simulink model "ALL_JP360_DBW_V6_5_1103"  (R2022a)
settings: Solver=FixedStepAuto  StartTime=0.0  StopTime=inf  FixedStep=0.01  RelTol=1e-3  EnableMultiTasking=on
model workspace (MAT data in the model file):
  g = 9.8
undefined symbols (not defined in the file or in its folder): canChannel, delta_v_p, IPM_Line_C0, IPM_Line_C1, IPM_Line_C2, IPM_Line_C3, M, M_p, MRR_ObjDistX, MRR_ObjDistY, MRR_ObjFusionCamID, MRR_ObjFusionSig, MRR_ObjID, MRR_ObjRelVelX, MRR_ObjRelVelY, MRR_ObjType, MRR_ObjUpdFlg, none, obj_vaild, untracktime, V, videoinput
libraries: canfdmsglib x230, canfdlib x76, slpidlib x24, simulink x18, dspstat3 x14, ctrlSharedLib x1, simulink_extras x1, imaqlib x1, realtime_pacer_lib x1, dspvision x1, visionsinks x1
(part 47 of 55)

== system ALL_JP360_DBW_V6_5_1103/MsgFromCAN/VR_ADCU_MsgFromCAN/VR_ADCU_MRR_Obj_13_14_0x696 ==
  VR_ADCU_MRR_Obj_13_14_0x696FromInData : Inport  OutDataTypeStr=Bus:CAN_FD_MESSAGE_BUS
  Bus Creator : BusCreator  Inputs=30  OutDataTypeStr=Bus:VR_ADCU_MRR_Obj_13_14_0x696  NonVirtualBus=on
  CAN FD Unpack : canfdmsglib/CAN FD Unpack  CANdbFile=HiFire_T360_P789_1R1V_Pri_Matrix_CAN_V2.3_20220810.dbc  MsgList=(none)  MsgName=MRR_Obj_13_14_0x696  ProtocolMode=CAN FD  MsgIDType=Standard (11-bit identifier)  MsgIdentifier=1686  MsgLength=32  SignalInfo={'MRR_ObjDistX_13','26','12','BE','unsigned','Standard','0','0.0625','0','0','254.9375';'MRR_ObjDistX_14','130','12','BE','unsigned','Standard','0','0.0625','0','0','254.9375';'MRR_ObjDistY_13','44','14','BE','unsigned','Standard','0','0.0078125','-64','-64','63.9922';'MRR_ObjDistY_14','148','14','BE','unsigned','Standard','0','0.0078125','-64','-64','63.9922';'MRR_ObjExistProb_13','11','5','BE','unsigned','Standard','0','0.03125','0','0','0.96875';'MRR_ObjExistProb_14','115','5','BE','unsigned','Standard','0','0.03125','0','0','0.96875';'MRR_ObjFusionCamID_13','208','8','BE','unsigned','Standard','0','1','0','0','255';'MRR_ObjFusionCamID_14','216','8','BE','unsigned','Standard','0','1','0','0','255';'MRR_ObjFusionSig_13','98','2','BE','unsigned','Standard','0','1','0','0','3';'MRR_ObjFusionSig_14','202','2','BE','unsigned','Standard','0','1','0','0','3';'MRR_ObjID_13','0','8','BE','unsigned','Standard','0','1','0','0','255';'MRR_ObjID_14','104','8','BE','unsigned','Standard','0','1','0','0','255';'MRR_ObjMovingSts_13','103','3','BE','unsigned','Standard','0','1','0','0','7';'MRR_ObjMovingSts_14','207','3','BE','unsigned','Standard','0','1','0','0','7';'MRR_ObjObstacleProb_13','22','5','BE','unsigned','Standard','0','0.03125','0','0','0.96875';'MRR_ObjObstacleProb_14','126','5','BE','unsigned','Standard','0','0.03125','0','0','0.96875';'MRR_ObjRelAccelX_13','72','10','BE','unsigned','Standard','0','0.03125','-16','-16','15.9688';'MRR_ObjRelAccelX_14','176','10','BE','unsigned','Standard','0','0.03125','-16','-16','15.9688';'MRR_ObjRelAccelY_13','94','10','BE','unsigned','Standard','0','0.03125','-16','-16','15.9688';'MRR_ObjRelAccelY_14','198','10','BE','unsigned','Standard','0','0.03125','-16','-16','15.9688';'MRR_ObjRelVelX_13','63','13','BE','unsigned','Standard','0','0.03125','-128','-128','127.9688';'MRR_ObjRelVelX_14','167','13','BE','unsigned','Standard','0','0.03125','-128','-128','127.9688';'MRR_ObjRelVelY_13','66','13','BE','unsigned','Standard','0','0.03125','-128','-128','127.9688';'MRR_ObjRelVelY_14','170','13','BE','unsigned','Standard','0','0.03125','-128','-128','127.9688';'MRR_ObjType_13','90','4','BE','unsigned','Standard','0','1','0','0','15';'MRR_ObjType_14','194','4','BE','unsigned','Standard','0','1','0','0','15';'MRR_ObjUpdFlg_13','100','3','BE','unsigned','Standard','0','1','0','0','7';'MRR_ObjUpdFlg_14','204','3','BE','unsigned','Standard','0','1','0','0','7';'MRR_Obj_13_14_Checksum','248','16','BE','unsigned','Standard','0','1','0','0','65535';'MRR_Obj_13_14_MsgCounter','232','4','BE','unsigned','Standard','0','1','0','0','15'}  IDPort=off  TimestampPort=off  ErrorPort=off  RemotePort=off  LengthPort=off  StatusPort=off  BRSPort=off  ESIPort=off  DLCPort=off  ApplyMinMax=off
      settings: SourceProductBaseCode=ME,XP,VN  DataFormat=CANdb specified signals
  Data Type Conversion{1..6,15..24} (16 alike) : DataTypeConversion  OutDataTypeStr=single  SaturateOnIntegerOverflow=off  RndMeth=Floor
  Data Type Conversion{9..10,13..14,25..28,30} (9 alike) : DataTypeConversion  OutDataTypeStr=int8  SaturateOnIntegerOverflow=off  RndMeth=Floor
  Data Type Conversion{7..8,11..12} (4 alike) : DataTypeConversion  OutDataTypeStr=uint8  SaturateOnIntegerOverflow=off  RndMeth=Floor
  Data Type Conversion29 : DataTypeConversion  OutDataTypeStr=uint16  SaturateOnIntegerOverflow=off  RndMeth=Floor
  VR_ADCU_MRR_Obj_13_14_0x696FromOutData : Outport  OutDataTypeStr=Bus:VR_ADCU_MRR_Obj_13_14_0x696
  wires:
  CAN FD Unpack/1 -> Data Type Conversion1/1
  CAN FD Unpack/2 -> Data Type Conversion2/1
  CAN FD Unpack/3 -> Data Type Conversion3/1
  CAN FD Unpack/4 -> Data Type Conversion4/1
  CAN FD Unpack/5 -> Data Type Conversion5/1
  CAN FD Unpack/6 -> Data Type Conversion6/1
  CAN FD Unpack/7 -> Data Type Conversion7/1
  CAN FD Unpack/8 -> Data Type Conversion8/1
  CAN FD Unpack/9 -> Data Type Conversion9/1
  CAN FD Unpack/10 -> Data Type Conversion10/1
  CAN FD Unpack/11 -> Data Type Conversion11/1
  CAN FD Unpack/12 -> Data Type Conversion12/1
  CAN FD Unpack/13 -> Data Type Conversion13/1
  CAN FD Unpack/14 -> Data Type Conversion14/1
  CAN FD Unpack/15 -> Data Type Conversion15/1
  CAN FD Unpack/16 -> Data Type Conversion16/1
  CAN FD Unpack/17 -> Data Type Conversion17/1
  CAN FD Unpack/18 -> Data Type Conversion18/1
  CAN FD Unpack/19 -> Data Type Conversion19/1
  CAN FD Unpack/20 -> Data Type Conversion20/1
  CAN FD Unpack/21 -> Data Type Conversion21/1
  CAN FD Unpack/22 -> Data Type Conversion22/1
  CAN FD Unpack/23 -> Data Type Conversion23/1
  CAN FD Unpack/24 -> Data Type Conversion24/1
  CAN FD Unpack/25 -> Data Type Conversion25/1
  CAN FD Unpack/26 -> Data Type Conversion26/1
  CAN FD Unpack/27 -> Data Type Conversion27/1
  CAN FD Unpack/28 -> Data Type Conversion28/1
  CAN FD Unpack/29 -> Data Type Conversion29/1
  CAN FD Unpack/30 -> Data Type Conversion30/1
  Data Type Conversion1/1 -> Bus Creator/1  "MRR_ObjDistX_13"
  Data Type Conversion2/1 -> Bus Creator/2  "MRR_ObjDistX_14"
  Data Type Conversion3/1 -> Bus Creator/3  "MRR_ObjDistY_13"
  Data Type Conversion4/1 -> Bus Creator/4  "MRR_ObjDistY_14"
  Data Type Conversion5/1 -> Bus Creator/5  "MRR_ObjExistProb_13"
  Data Type Conversion6/1 -> Bus Creator/6  "MRR_ObjExistProb_14"
  Data Type Conversion7/1 -> Bus Creator/7  "MRR_ObjFusionCamID_13"
  Data Type Conversion8/1 -> Bus Creator/8  "MRR_ObjFusionCamID_14"
  Data Type Conversion9/1 -> Bus Creator/9  "MRR_ObjFusionSig_13"
  Data Type Conversion10/1 -> Bus Creator/10  "MRR_ObjFusionSig_14"
  Data Type Conversion11/1 -> Bus Creator/11  "MRR_ObjID_13"
  Data Type Conversion12/1 -> Bus Creator/12  "MRR_ObjID_14"
  Data Type Conversion13/1 -> Bus Creator/13  "MRR_ObjMovingSts_13"
  Data Type Conversion14/1 -> Bus Creator/14  "MRR_ObjMovingSts_14"
  Data Type Conversion15/1 -> Bus Creator/15  "MRR_ObjObstacleProb_13"
  Data Type Conversion16/1 -> Bus Creator/16  "MRR_ObjObstacleProb_14"
  Data Type Conversion17/1 -> Bus Creator/17  "MRR_ObjRelAccelX_13"
  Data Type Conversion18/1 -> Bus Creator/18  "MRR_ObjRelAccelX_14"
  Data Type Conversion19/1 -> Bus Creator/19  "MRR_ObjRelAccelY_13"
  Data Type Conversion20/1 -> Bus Creator/20  "MRR_ObjRelAccelY_14"
  Data Type Conversion21/1 -> Bus Creator/21  "MRR_ObjRelVelX_13"
  Data Type Conversion22/1 -> Bus Creator/22  "MRR_ObjRelVelX_14"
  Data Type Conversion23/1 -> Bus Creator/23  "MRR_ObjRelVelY_13"
  Data Type Conversion24/1 -> Bus Creator/24  "MRR_ObjRelVelY_14"
  Data Type Conversion25/1 -> Bus Creator/25  "MRR_ObjType_13"
  Data Type Conversion26/1 -> Bus Creator/26  "MRR_ObjType_14"
  Data Type Conversion27/1 -> Bus Creator/27  "MRR_ObjUpdFlg_13"
  Data Type Conversion28/1 -> Bus Creator/28  "MRR_ObjUpdFlg_14"
  Data Type Conversion29/1 -> Bus Creator/29  "MRR_Obj_13_14_Checksum"
  Data Type Conversion30/1 -> Bus Creator/30  "MRR_Obj_13_14_MsgCounter"
  Bus Creator/1 -> VR_ADCU_MRR_Obj_13_14_0x696FromOutData/1  "VR_ADCU_MRR_Obj_13_14_0x696FromOutData"
  VR_ADCU_MRR_Obj_13_14_0x696FromInData/1 -> CAN FD Unpack/1  "VR_ADCU_MRR_Obj_13_14_0x696FromInData"

== system ALL_JP360_DBW_V6_5_1103/MsgFromCAN/VR_ADCU_MsgFromCAN/VR_ADCU_MRR_Obj_15_16_0x697 ==
  VR_ADCU_MRR_Obj_15_16_0x697FromInData : Inport  OutDataTypeStr=Bus:CAN_FD_MESSAGE_BUS
  Bus Creator : BusCreator  Inputs=30  OutDataTypeStr=Bus:VR_ADCU_MRR_Obj_15_16_0x697  NonVirtualBus=on
  CAN FD Unpack : canfdmsglib/CAN FD Unpack  CANdbFile=HiFire_T360_P789_1R1V_Pri_Matrix_CAN_V2.3_20220810.dbc  MsgList=(none)  MsgName=MRR_Obj_15_16_0x697  ProtocolMode=CAN FD  MsgIDType=Standard (11-bit identifier)  MsgIdentifier=1687  MsgLength=32  SignalInfo={'MRR_ObjDistX_15','26','12','BE','unsigned','Standard','0','0.0625','0','0','254.9375';'MRR_ObjDistX_16','130','12','BE','unsigned','Standard','0','0.0625','0','0','254.9375';'MRR_ObjDistY_15','44','14','BE','unsigned','Standard','0','0.0078125','-64','-64','63.9922';'MRR_ObjDistY_16','148','14','BE','unsigned','Standard','0','0.0078125','-64','-64','63.9922';'MRR_ObjExistProb_15','11','5','BE','unsigned','Standard','0','0.03125','0','0','0.96875';'MRR_ObjExistProb_16','115','5','BE','unsigned','Standard','0','0.03125','0','0','0.96875';'MRR_ObjFusionCamID_15','208','8','BE','unsigned','Standard','0','1','0','0','255';'MRR_ObjFusionCamID_16','216','8','BE','unsigned','Standard','0','1','0','0','255';'MRR_ObjFusionSig_15','98','2','BE','unsigned','Standard','0','1','0','0','3';'MRR_ObjFusionSig_16','202','2','BE','unsigned','Standard','0','1','0','0','3';'MRR_ObjID_15','0','8','BE','unsigned','Standard','0','1','0','0','255';'MRR_ObjID_16','104','8','BE','unsigned','Standard','0','1','0','0','255';'MRR_ObjMovingSts_15','103','3','BE','unsigned','Standard','0','1','0','0','7';'MRR_ObjMovingSts_16','207','3','BE','unsigned','Standard','0','1','0','0','7';'MRR_ObjObstacleProb_15','22','5','BE','unsigned','Standard','0','0.03125','0','0','0.96875';'MRR_ObjObstacleProb_16','126','5','BE','unsigned','Standard','0','0.03125','0','0','0.96875';'MRR_ObjRelAccelX_15','72','10','BE','unsigned','Standard','0','0.03125','-16','-16','15.9688';'MRR_ObjRelAccelX_16','176','10','BE','unsigned','Standard','0','0.03125','-16','-16','15.9688';'MRR_ObjRelAccelY_15','94','10','BE','unsigned','Standard','0','0.03125','-16','-16','15.9688';'MRR_ObjRelAccelY_16','198','10','BE','unsigned','Standard','0','0.03125','-16','-16','15.9688';'MRR_ObjRelVelX_15','63','13','BE','unsigned','Standard','0','0.03125','-128','-128','127.9688';'MRR_ObjRelVelX_16','167','13','BE','unsigned','Standard','0','0.03125','-128','-128','127.9688';'MRR_ObjRelVelY_15','66','13','BE','unsigned','Standard','0','0.03125','-128','-128','127.9688';'MRR_ObjRelVelY_16','170','13','BE','unsigned','Standard','0','0.03125','-128','-128','127.9688';'MRR_ObjType_15','90','4','BE','unsigned','Standard','0','1','0','0','15';'MRR_ObjType_16','194','4','BE','unsigned','Standard','0','1','0','0','15';'MRR_ObjUpdFlg_15','100','3','BE','unsigned','Standard','0','1','0','0','7';'MRR_ObjUpdFlg_16','204','3','BE','unsigned','Standard','0','1','0','0','7';'MRR_Obj_15_16_Checksum','248','16','BE','unsigned','Standard','0','1','0','0','65535';'MRR_Obj_15_16_MsgCounter','232','4','BE','unsigned','Standard','0','1','0','0','15'}  IDPort=off  TimestampPort=off  ErrorPort=off  RemotePort=off  LengthPort=off  StatusPort=off  BRSPort=off  ESIPort=off  DLCPort=off  ApplyMinMax=off
      settings: SourceProductBaseCode=ME,XP,VN  DataFormat=CANdb specified signals
  Data Type Conversion{1..6,15..24} (16 alike) : DataTypeConversion  OutDataTypeStr=single  SaturateOnIntegerOverflow=off  RndMeth=Floor
  Data Type Conversion{9..10,13..14,25..28,30} (9 alike) : DataTypeConversion  OutDataTypeStr=int8  SaturateOnIntegerOverflow=off  RndMeth=Floor
  Data Type Conversion{7..8,11..12} (4 alike) : DataTypeConversion  OutDataTypeStr=uint8  SaturateOnIntegerOverflow=off  RndMeth=Floor
  Data Type Conversion29 : DataTypeConversion  OutDataTypeStr=uint16  SaturateOnIntegerOverflow=off  RndMeth=Floor
  VR_ADCU_MRR_Obj_15_16_0x697FromOutData : Outport  OutDataTypeStr=Bus:VR_ADCU_MRR_Obj_15_16_0x697
  wires:
  CAN FD Unpack/1 -> Data Type Conversion1/1
  CAN FD Unpack/2 -> Data Type Conversion2/1
  CAN FD Unpack/3 -> Data Type Conversion3/1
  CAN FD Unpack/4 -> Data Type Conversion4/1
  CAN FD Unpack/5 -> Data Type Conversion5/1
  CAN FD Unpack/6 -> Data Type Conversion6/1
  CAN FD Unpack/7 -> Data Type Conversion7/1
  CAN FD Unpack/8 -> Data Type Conversion8/1
  CAN FD Unpack/9 -> Data Type Conversion9/1
  CAN FD Unpack/10 -> Data Type Conversion10/1
  CAN FD Unpack/11 -> Data Type Conversion11/1
  CAN FD Unpack/12 -> Data Type Conversion12/1
  CAN FD Unpack/13 -> Data Type Conversion13/1
  CAN FD Unpack/14 -> Data Type Conversion14/1
  CAN FD Unpack/15 -> Data Type Conversion15/1
  CAN FD Unpack/16 -> Data Type Conversion16/1
  CAN FD Unpack/17 -> Data Type Conversion17/1
  CAN FD Unpack/18 -> Data Type Conversion18/1
  CAN FD Unpack/19 -> Data Type Conversion19/1
  CAN FD Unpack/20 -> Data Type Conversion20/1
  CAN FD Unpack/21 -> Data Type Conversion21/1
  CAN FD Unpack/22 -> Data Type Conversion22/1
  CAN FD Unpack/23 -> Data Type Conversion23/1
  CAN FD Unpack/24 -> Data Type Conversion24/1
  CAN FD Unpack/25 -> Data Type Conversion25/1
  CAN FD Unpack/26 -> Data Type Conversion26/1
  CAN FD Unpack/27 -> Data Type Conversion27/1
  CAN FD Unpack/28 -> Data Type Conversion28/1
  CAN FD Unpack/29 -> Data Type Conversion29/1
  CAN FD Unpack/30 -> Data Type Conversion30/1
  Data Type Conversion1/1 -> Bus Creator/1  "MRR_ObjDistX_15"
  Data Type Conversion2/1 -> Bus Creator/2  "MRR_ObjDistX_16"
  Data Type Conversion3/1 -> Bus Creator/3  "MRR_ObjDistY_15"
  Data Type Conversion4/1 -> Bus Creator/4  "MRR_ObjDistY_16"
  Data Type Conversion5/1 -> Bus Creator/5  "MRR_ObjExistProb_15"
  Data Type Conversion6/1 -> Bus Creator/6  "MRR_ObjExistProb_16"
  Data Type Conversion7/1 -> Bus Creator/7  "MRR_ObjFusionCamID_15"
  Data Type Conversion8/1 -> Bus Creator/8  "MRR_ObjFusionCamID_16"
  Data Type Conversion9/1 -> Bus Creator/9  "MRR_ObjFusionSig_15"
  Data Type Conversion10/1 -> Bus Creator/10  "MRR_ObjFusionSig_16"
  Data Type Conversion11/1 -> Bus Creator/11  "MRR_ObjID_15"
  Data Type Conversion12/1 -> Bus Creator/12  "MRR_ObjID_16"
  Data Type Conversion13/1 -> Bus Creator/13  "MRR_ObjMovingSts_15"
  Data Type Conversion14/1 -> Bus Creator/14  "MRR_ObjMovingSts_16"
  Data Type Conversion15/1 -> Bus Creator/15  "MRR_ObjObstacleProb_15"
  Data Type Conversion16/1 -> Bus Creator/16  "MRR_ObjObstacleProb_16"
  Data Type Conversion17/1 -> Bus Creator/17  "MRR_ObjRelAccelX_15"
  Data Type Conversion18/1 -> Bus Creator/18  "MRR_ObjRelAccelX_16"
  Data Type Conversion19/1 -> Bus Creator/19  "MRR_ObjRelAccelY_15"
  Data Type Conversion20/1 -> Bus Creator/20  "MRR_ObjRelAccelY_16"
  Data Type Conversion21/1 -> Bus Creator/21  "MRR_ObjRelVelX_15"
  Data Type Conversion22/1 -> Bus Creator/22  "MRR_ObjRelVelX_16"
  Data Type Conversion23/1 -> Bus Creator/23  "MRR_ObjRelVelY_15"
  Data Type Conversion24/1 -> Bus Creator/24  "MRR_ObjRelVelY_16"
  Data Type Conversion25/1 -> Bus Creator/25  "MRR_ObjType_15"
  Data Type Conversion26/1 -> Bus Creator/26  "MRR_ObjType_16"
  Data Type Conversion27/1 -> Bus Creator/27  "MRR_ObjUpdFlg_15"
  Data Type Conversion28/1 -> Bus Creator/28  "MRR_ObjUpdFlg_16"
  Data Type Conversion29/1 -> Bus Creator/29  "MRR_Obj_15_16_Checksum"
  Data Type Conversion30/1 -> Bus Creator/30  "MRR_Obj_15_16_MsgCounter"
  Bus Creator/1 -> VR_ADCU_MRR_Obj_15_16_0x697FromOutData/1  "VR_ADCU_MRR_Obj_15_16_0x697FromOutData"
  VR_ADCU_MRR_Obj_15_16_0x697FromInData/1 -> CAN FD Unpack/1  "VR_ADCU_MRR_Obj_15_16_0x697FromInData"

== system ALL_JP360_DBW_V6_5_1103/MsgFromCAN/VR_ADCU_MsgFromCAN/VR_ADCU_MRR_Obj_17_18_0x698 ==
  VR_ADCU_MRR_Obj_17_18_0x698FromInData : Inport  OutDataTypeStr=Bus:CAN_FD_MESSAGE_BUS
  Bus Creator : BusCreator  Inputs=30  OutDataTypeStr=Bus:VR_ADCU_MRR_Obj_17_18_0x698  NonVirtualBus=on
  CAN FD Unpack : canfdmsglib/CAN FD Unpack  CANdbFile=HiFire_T360_P789_1R1V_Pri_Matrix_CAN_V2.3_20220810.dbc  MsgList=(none)  MsgName=MRR_Obj_17_18_0x698  ProtocolMode=CAN FD  MsgIDType=Standard (11-bit identifier)  MsgIdentifier=1688  MsgLength=32  SignalInfo={'MRR_ObjDistX_17','26','12','BE','unsigned','Standard','0','0.0625','0','0','254.9375';'MRR_ObjDistX_18','130','12','BE','unsigned','Standard','0','0.0625','0','0','254.9375';'MRR_ObjDistY_17','44','14','BE','unsigned','Standard','0','0.0078125','-64','-64','63.9922';'MRR_ObjDistY_18','148','14','BE','unsigned','Standard','0','0.0078125','-64','-64','63.9922';'MRR_ObjExistProb_17','11','5','BE','unsigned','Standard','0','0.03125','0','0','0.96875';'MRR_ObjExistProb_18','115','5','BE','unsigned','Standard','0','0.03125','0','0','0.96875';'MRR_ObjFusionCamID_17','208','8','BE','unsigned','Standard','0','1','0','0','255';'MRR_ObjFusionCamID_18','216','8','BE','unsigned','Standard','0','1','0','0','255';'MRR_ObjFusionSig_17','98','2','BE','unsigned','Standard','0','1','0','0','3';'MRR_ObjFusionSig_18','202','2','BE','unsigned','Standard','0','1','0','0','3';'MRR_ObjID_17','0','8','BE','unsigned','Standard','0','1','0','0','255';'MRR_ObjID_18','104','8','BE','unsigned','Standard','0','1','0','0','255';'MRR_ObjMovingSts_17','103','3','BE','unsigned','Standard','0','1','0','0','7';'MRR_ObjMovingSts_18','207','3','BE','unsigned','Standard','0','1','0','0','7';'MRR_ObjObstacleProb_17','22','5','BE','unsigned','Standard','0','0.03125','0','0','0.96875';'MRR_ObjObstacleProb_18','126','5','BE','unsigned','Standard','0','0.03125','0','0','0.96875';'MRR_ObjRelAccelX_17','72','10','BE','unsigned','Standard','0','0.03125','-16','-16','15.9688';'MRR_ObjRelAccelX_18','176','10','BE','unsigned','Standard','0','0.03125','-16','-16','15.9688';'MRR_ObjRelAccelY_17','94','10','BE','unsigned','Standard','0','0.03125','-16','-16','15.9688';'MRR_ObjRelAccelY_18','198','10','BE','unsigned','Standard','0','0.03125','-16','-16','15.9688';'MRR_ObjRelVelX_17','63','13','BE','unsigned','Standard','0','0.03125','-128','-128','127.9688';'MRR_ObjRelVelX_18','167','13','BE','unsigned','Standard','0','0.03125','-128','-128','127.9688';'MRR_ObjRelVelY_17','66','13','BE','unsigned','Standard','0','0.03125','-128','-128','127.9688';'MRR_ObjRelVelY_18','170','13','BE','unsigned','Standard','0','0.03125','-128','-128','127.9688';'MRR_ObjType_17','90','4','BE','unsigned','Standard','0','1','0','0','15';'MRR_ObjType_18','194','4','BE','unsigned','Standard','0','1','0','0','15';'MRR_ObjUpdFlg_17','100','3','BE','unsigned','Standard','0','1','0','0','7';'MRR_ObjUpdFlg_18','204','3','BE','unsigned','Standard','0','1','0','0','7';'MRR_Obj_17_18_Checksum','248','16','BE','unsigned','Standard','0','1','0','0','65535';'MRR_Obj_17_18_MsgCounter','232','4','BE','unsigned','Standard','0','1','0','0','15'}  IDPort=off  TimestampPort=off  ErrorPort=off  RemotePort=off  LengthPort=off  StatusPort=off  BRSPort=off  ESIPort=off  DLCPort=off  ApplyMinMax=off
      settings: SourceProductBaseCode=ME,XP,VN  DataFormat=CANdb specified signals
  Data Type Conversion{1..6,15..24} (16 alike) : DataTypeConversion  OutDataTypeStr=single  SaturateOnIntegerOverflow=off  RndMeth=Floor
  Data Type Conversion{9..10,13..14,25..28,30} (9 alike) : DataTypeConversion  OutDataTypeStr=int8  SaturateOnIntegerOverflow=off  RndMeth=Floor
  Data Type Conversion{7..8,11..12} (4 alike) : DataTypeConversion  OutDataTypeStr=uint8  SaturateOnIntegerOverflow=off  RndMeth=Floor
  Data Type Conversion29 : DataTypeConversion  OutDataTypeStr=uint16  SaturateOnIntegerOverflow=off  RndMeth=Floor
  VR_ADCU_MRR_Obj_17_18_0x698FromOutData : Outport  OutDataTypeStr=Bus:VR_ADCU_MRR_Obj_17_18_0x698
  wires:
  CAN FD Unpack/1 -> Data Type Conversion1/1
  CAN FD Unpack/2 -> Data Type Conversion2/1
  CAN FD Unpack/3 -> Data Type Conversion3/1
  CAN FD Unpack/4 -> Data Type Conversion4/1
  CAN FD Unpack/5 -> Data Type Conversion5/1
  CAN FD Unpack/6 -> Data Type Conversion6/1
  CAN FD Unpack/7 -> Data Type Conversion7/1
  CAN FD Unpack/8 -> Data Type Conversion8/1
  CAN FD Unpack/9 -> Data Type Conversion9/1
  CAN FD Unpack/10 -> Data Type Conversion10/1
  CAN FD Unpack/11 -> Data Type Conversion11/1
  CAN FD Unpack/12 -> Data Type Conversion12/1
  CAN FD Unpack/13 -> Data Type Conversion13/1
  CAN FD Unpack/14 -> Data Type Conversion14/1
  CAN FD Unpack/15 -> Data Type Conversion15/1
  CAN FD Unpack/16 -> Data Type Conversion16/1
  CAN FD Unpack/17 -> Data Type Conversion17/1
  CAN FD Unpack/18 -> Data Type Conversion18/1
  CAN FD Unpack/19 -> Data Type Conversion19/1
  CAN FD Unpack/20 -> Data Type Conversion20/1
  CAN FD Unpack/21 -> Data Type Conversion21/1
  CAN FD Unpack/22 -> Data Type Conversion22/1
  CAN FD Unpack/23 -> Data Type Conversion23/1
  CAN FD Unpack/24 -> Data Type Conversion24/1
  CAN FD Unpack/25 -> Data Type Conversion25/1
  CAN FD Unpack/26 -> Data Type Conversion26/1
  CAN FD Unpack/27 -> Data Type Conversion27/1
  CAN FD Unpack/28 -> Data Type Conversion28/1
  CAN FD Unpack/29 -> Data Type Conversion29/1
  CAN FD Unpack/30 -> Data Type Conversion30/1
  Data Type Conversion1/1 -> Bus Creator/1  "MRR_ObjDistX_17"
  Data Type Conversion2/1 -> Bus Creator/2  "MRR_ObjDistX_18"
  Data Type Conversion3/1 -> Bus Creator/3  "MRR_ObjDistY_17"
  Data Type Conversion4/1 -> Bus Creator/4  "MRR_ObjDistY_18"
  Data Type Conversion5/1 -> Bus Creator/5  "MRR_ObjExistProb_17"
  Data Type Conversion6/1 -> Bus Creator/6  "MRR_ObjExistProb_18"
  Data Type Conversion7/1 -> Bus Creator/7  "MRR_ObjFusionCamID_17"
  Data Type Conversion8/1 -> Bus Creator/8  "MRR_ObjFusionCamID_18"
  Data Type Conversion9/1 -> Bus Creator/9  "MRR_ObjFusionSig_17"
  Data Type Conversion10/1 -> Bus Creator/10  "MRR_ObjFusionSig_18"
  Data Type Conversion11/1 -> Bus Creator/11  "MRR_ObjID_17"
  Data Type Conversion12/1 -> Bus Creator/12  "MRR_ObjID_18"
  Data Type Conversion13/1 -> Bus Creator/13  "MRR_ObjMovingSts_17"
  Data Type Conversion14/1 -> Bus Creator/14  "MRR_ObjMovingSts_18"
  Data Type Conversion15/1 -> Bus Creator/15  "MRR_ObjObstacleProb_17"
  Data Type Conversion16/1 -> Bus Creator/16  "MRR_ObjObstacleProb_18"
  Data Type Conversion17/1 -> Bus Creator/17  "MRR_ObjRelAccelX_17"
  Data Type Conversion18/1 -> Bus Creator/18  "MRR_ObjRelAccelX_18"
  Data Type Conversion19/1 -> Bus Creator/19  "MRR_ObjRelAccelY_17"
  Data Type Conversion20/1 -> Bus Creator/20  "MRR_ObjRelAccelY_18"
  Data Type Conversion21/1 -> Bus Creator/21  "MRR_ObjRelVelX_17"
  Data Type Conversion22/1 -> Bus Creator/22  "MRR_ObjRelVelX_18"
  Data Type Conversion23/1 -> Bus Creator/23  "MRR_ObjRelVelY_17"
  Data Type Conversion24/1 -> Bus Creator/24  "MRR_ObjRelVelY_18"
  Data Type Conversion25/1 -> Bus Creator/25  "MRR_ObjType_17"
  Data Type Conversion26/1 -> Bus Creator/26  "MRR_ObjType_18"
  Data Type Conversion27/1 -> Bus Creator/27  "MRR_ObjUpdFlg_17"
  Data Type Conversion28/1 -> Bus Creator/28  "MRR_ObjUpdFlg_18"
  Data Type Conversion29/1 -> Bus Creator/29  "MRR_Obj_17_18_Checksum"
  Data Type Conversion30/1 -> Bus Creator/30  "MRR_Obj_17_18_MsgCounter"
  Bus Creator/1 -> VR_ADCU_MRR_Obj_17_18_0x698FromOutData/1  "VR_ADCU_MRR_Obj_17_18_0x698FromOutData"
  VR_ADCU_MRR_Obj_17_18_0x698FromInData/1 -> CAN FD Unpack/1  "VR_ADCU_MRR_Obj_17_18_0x698FromInData"

== system ALL_JP360_DBW_V6_5_1103/MsgFromCAN/VR_ADCU_MsgFromCAN/VR_ADCU_MRR_Obj_19_20_0x699 ==
  VR_ADCU_MRR_Obj_19_20_0x699FromInData : Inport  OutDataTypeStr=Bus:CAN_FD_MESSAGE_BUS
  Bus Creator : BusCreator  Inputs=30  OutDataTypeStr=Bus:VR_ADCU_MRR_Obj_19_20_0x699  NonVirtualBus=on
  CAN FD Unpack : canfdmsglib/CAN FD Unpack  CANdbFile=HiFire_T360_P789_1R1V_Pri_Matrix_CAN_V2.3_20220810.dbc  MsgList=(none)  MsgName=MRR_Obj_19_20_0x699  ProtocolMode=CAN FD  MsgIDType=Standard (11-bit identifier)  MsgIdentifier=1689  MsgLength=32  SignalInfo={'MRR_ObjDistX_19','26','12','BE','unsigned','Standard','0','0.0625','0','0','254.9375';'MRR_ObjDistX_20','130','12','BE','unsigned','Standard','0','0.0625','0','0','254.9375';'MRR_ObjDistY_19','44','14','BE','unsigned','Standard','0','0.0078125','-64','-64','63.9922';'MRR_ObjDistY_20','148','14','BE','unsigned','Standard','0','0.0078125','-64','-64','63.9922';'MRR_ObjExistProb_19','11','5','BE','unsigned','Standard','0','0.03125','0','0','0.96875';'MRR_ObjExistProb_20','115','5','BE','unsigned','Standard','0','0.03125','0','0','0.96875';'MRR_ObjFusionCamID_19','208','8','BE','unsigned','Standard','0','1','0','0','255';'MRR_ObjFusionCamID_20','216','8','BE','unsigned','Standard','0','1','0','0','255';'MRR_ObjFusionSig_19','98','2','BE','unsigned','Standard','0','1','0','0','3';'MRR_ObjFusionSig_20','202','2','BE','unsigned','Standard','0','1','0','0','3';'MRR_ObjID_19','0','8','BE','unsigned','Standard','0','1','0','0','255';'MRR_ObjID_20','104','8','BE','unsigned','Standard','0','1','0','0','255';'MRR_ObjMovingSts_19','103','3','BE','unsigned','Standard','0','1','0','0','7';'MRR_ObjMovingSts_20','207','3','BE','unsigned','Standard','0','1','0','0','7';'MRR_ObjObstacleProb_19','22','5','BE','unsigned','Standard','0','0.03125','0','0','0.96875';'MRR_ObjObstacleProb_20','126','5','BE','unsigned','Standard','0','0.03125','0','0','0.96875';'MRR_ObjRelAccelX_19','72','10','BE','unsigned','Standard','0','0.03125','-16','-16','15.9688';'MRR_ObjRelAccelX_20','176','10','BE','unsigned','Standard','0','0.03125','-16','-16','15.9688';'MRR_ObjRelAccelY_19','94','10','BE','unsigned','Standard','0','0.03125','-16','-16','15.9688';'MRR_ObjRelAccelY_20','198','10','BE','unsigned','Standard','0','0.03125','-16','-16','15.9688';'MRR_ObjRelVelX_19','63','13','BE','unsigned','Standard','0','0.03125','-128','-128','127.9688';'MRR_ObjRelVelX_20','167','13','BE','unsigned','Standard','0','0.03125','-128','-128','127.9688';'MRR_ObjRelVelY_19','66','13','BE','unsigned','Standard','0','0.03125','-128','-128','127.9688';'MRR_ObjRelVelY_20','170','13','BE','unsigned','Standard','0','0.03125','-128','-128','127.9688';'MRR_ObjType_19','90','4','BE','unsigned','Standard','0','1','0','0','15';'MRR_ObjType_20','194','4','BE','unsigned','Standard','0','1','0','0','15';'MRR_ObjUpdFlg_19','100','3','BE','unsigned','Standard','0','1','0','0','7';'MRR_ObjUpdFlg_20','204','3','BE','unsigned','Standard','0','1','0','0','7';'MRR_Obj_19_20_Checksum','248','16','BE','unsigned','Standard','0','1','0','0','65535';'MRR_Obj_19_20_MsgCounter','232','4','BE','unsigned','Standard','0','1','0','0','15'}  IDPort=off  TimestampPort=off  ErrorPort=off  RemotePort=off  LengthPort=off  StatusPort=off  BRSPort=off  ESIPort=off  DLCPort=off  ApplyMinMax=off
      settings: SourceProductBaseCode=ME,XP,VN  DataFormat=CANdb specified signals
  Data Type Conversion{1..6,15..24} (16 alike) : DataTypeConversion  OutDataTypeStr=single  SaturateOnIntegerOverflow=off  RndMeth=Floor
  Data Type Conversion{9..10,13..14,25..28,30} (9 alike) : DataTypeConversion  OutDataTypeStr=int8  SaturateOnIntegerOverflow=off  RndMeth=Floor
  Data Type Conversion{7..8,11..12} (4 alike) : DataTypeConversion  OutDataTypeStr=uint8  SaturateOnIntegerOverflow=off  RndMeth=Floor
  Data Type Conversion29 : DataTypeConversion  OutDataTypeStr=uint16  SaturateOnIntegerOverflow=off  RndMeth=Floor
  VR_ADCU_MRR_Obj_19_20_0x699FromOutData : Outport  OutDataTypeStr=Bus:VR_ADCU_MRR_Obj_19_20_0x699
  wires:
  CAN FD Unpack/1 -> Data Type Conversion1/1
  CAN FD Unpack/2 -> Data Type Conversion2/1
  CAN FD Unpack/3 -> Data Type Conversion3/1
  CAN FD Unpack/4 -> Data Type Conversion4/1
  CAN FD Unpack/5 -> Data Type Conversion5/1
  CAN FD Unpack/6 -> Data Type Conversion6/1
  CAN FD Unpack/7 -> Data Type Conversion7/1
  CAN FD Unpack/8 -> Data Type Conversion8/1
  CAN FD Unpack/9 -> Data Type Conversion9/1
  CAN FD Unpack/10 -> Data Type Conversion10/1
  CAN FD Unpack/11 -> Data Type Conversion11/1
  CAN FD Unpack/12 -> Data Type Conversion12/1
  CAN FD Unpack/13 -> Data Type Conversion13/1
  CAN FD Unpack/14 -> Data Type Conversion14/1
  CAN FD Unpack/15 -> Data Type Conversion15/1
  CAN FD Unpack/16 -> Data Type Conversion16/1
  CAN FD Unpack/17 -> Data Type Conversion17/1
  CAN FD Unpack/18 -> Data Type Conversion18/1
  CAN FD Unpack/19 -> Data Type Conversion19/1
  CAN FD Unpack/20 -> Data Type Conversion20/1
  CAN FD Unpack/21 -> Data Type Conversion21/1
  CAN FD Unpack/22 -> Data Type Conversion22/1
  CAN FD Unpack/23 -> Data Type Conversion23/1
  CAN FD Unpack/24 -> Data Type Conversion24/1
  CAN FD Unpack/25 -> Data Type Conversion25/1
  CAN FD Unpack/26 -> Data Type Conversion26/1
  CAN FD Unpack/27 -> Data Type Conversion27/1
  CAN FD Unpack/28 -> Data Type Conversion28/1
  CAN FD Unpack/29 -> Data Type Conversion29/1
  CAN FD Unpack/30 -> Data Type Conversion30/1
  Data Type Conversion1/1 -> Bus Creator/1  "MRR_ObjDistX_19"
  Data Type Conversion2/1 -> Bus Creator/2  "MRR_ObjDistX_20"
  Data Type Conversion3/1 -> Bus Creator/3  "MRR_ObjDistY_19"
  Data Type Conversion4/1 -> Bus Creator/4  "MRR_ObjDistY_20"
  Data Type Conversion5/1 -> Bus Creator/5  "MRR_ObjExistProb_19"
  Data Type Conversion6/1 -> Bus Creator/6  "MRR_ObjExistProb_20"
  Data Type Conversion7/1 -> Bus Creator/7  "MRR_ObjFusionCamID_19"
  Data Type Conversion8/1 -> Bus Creator/8  "MRR_ObjFusionCamID_20"
  Data Type Conversion9/1 -> Bus Creator/9  "MRR_ObjFusionSig_19"
  Data Type Conversion10/1 -> Bus Creator/10  "MRR_ObjFusionSig_20"
  Data Type Conversion11/1 -> Bus Creator/11  "MRR_ObjID_19"
  Data Type Conversion12/1 -> Bus Creator/12  "MRR_ObjID_20"
  Data Type Conversion13/1 -> Bus Creator/13  "MRR_ObjMovingSts_19"
  Data Type Conversion14/1 -> Bus Creator/14  "MRR_ObjMovingSts_20"
  Data Type Conversion15/1 -> Bus Creator/15  "MRR_ObjObstacleProb_19"
  Data Type Conversion16/1 -> Bus Creator/16  "MRR_ObjObstacleProb_20"
  Data Type Conversion17/1 -> Bus Creator/17  "MRR_ObjRelAccelX_19"
  Data Type Conversion18/1 -> Bus Creator/18  "MRR_ObjRelAccelX_20"
  Data Type Conversion19/1 -> Bus Creator/19  "MRR_ObjRelAccelY_19"
  Data Type Conversion20/1 -> Bus Creator/20  "MRR_ObjRelAccelY_20"
  Data Type Conversion21/1 -> Bus Creator/21  "MRR_ObjRelVelX_19"
  Data Type Conversion22/1 -> Bus Creator/22  "MRR_ObjRelVelX_20"
  Data Type Conversion23/1 -> Bus Creator/23  "MRR_ObjRelVelY_19"
  Data Type Conversion24/1 -> Bus Creator/24  "MRR_ObjRelVelY_20"
  Data Type Conversion25/1 -> Bus Creator/25  "MRR_ObjType_19"
  Data Type Conversion26/1 -> Bus Creator/26  "MRR_ObjType_20"
  Data Type Conversion27/1 -> Bus Creator/27  "MRR_ObjUpdFlg_19"
  Data Type Conversion28/1 -> Bus Creator/28  "MRR_ObjUpdFlg_20"
  Data Type Conversion29/1 -> Bus Creator/29  "MRR_Obj_19_20_Checksum"
  Data Type Conversion30/1 -> Bus Creator/30  "MRR_Obj_19_20_MsgCounter"
  Bus Creator/1 -> VR_ADCU_MRR_Obj_19_20_0x699FromOutData/1  "VR_ADCU_MRR_Obj_19_20_0x699FromOutData"
  VR_ADCU_MRR_Obj_19_20_0x699FromInData/1 -> CAN FD Unpack/1  "VR_ADCU_MRR_Obj_19_20_0x699FromInData"

== system ALL_JP360_DBW_V6_5_1103/MsgFromCAN/VR_ADCU_MsgFromCAN/VR_ADCU_MRR_Obj_21_22_0x69A ==
  VR_ADCU_MRR_Obj_21_22_0x69AFromInData : Inport  OutDataTypeStr=Bus:CAN_FD_MESSAGE_BUS
  Bus Creator : BusCreator  Inputs=30  OutDataTypeStr=Bus:VR_ADCU_MRR_Obj_21_22_0x69A  NonVirtualBus=on
  CAN FD Unpack : canfdmsglib/CAN FD Unpack  CANdbFile=HiFire_T360_P789_1R1V_Pri_Matrix_CAN_V2.3_20220810.dbc  MsgList=(none)  MsgName=MRR_Obj_21_22_0x69A  ProtocolMode=CAN FD  MsgIDType=Standard (11-bit identifier)  MsgIdentifier=1690  MsgLength=32  SignalInfo={'MRR_ObjDistX_21','26','12','BE','unsigned','Standard','0','0.0625','0','0','254.9375';'MRR_ObjDistX_22','130','12','BE','unsigned','Standard','0','0.0625','0','0','254.9375';'MRR_ObjDistY_21','44','14','BE','unsigned','Standard','0','0.0078125','-64','-64','63.9922';'MRR_ObjDistY_22','148','14','BE','unsigned','Standard','0','0.0078125','-64','-64','63.9922';'MRR_ObjExistProb_21','11','5','BE','unsigned','Standard','0','0.03125','0','0','0.96875';'MRR_ObjExistProb_22','115','5','BE','unsigned','Standard','0','0.03125','0','0','0.96875';'MRR_ObjFusionCamID_21','208','8','BE','unsigned','Standard','0','1','0','0','255';'MRR_ObjFusionCamID_22','216','8','BE','unsigned','Standard','0','1','0','0','255';'MRR_ObjFusionSig_21','98','2','BE','unsigned','Standard','0','1','0','0','3';'MRR_ObjFusionSig_22','202','2','BE','unsigned','Standard','0','1','0','0','3';'MRR_ObjID_21','0','8','BE','unsigned','Standard','0','1','0','0','255';'MRR_ObjID_22','104','8','BE','unsigned','Standard','0','1','0','0','255';'MRR_ObjMovingSts_21','103','3','BE','unsigned','Standard','0','1','0','0','7';'MRR_ObjMovingSts_22','207','3','BE','unsigned','Standard','0','1','0','0','7';'MRR_ObjObstacleProb_21','22','5','BE','unsigned','Standard','0','0.03125','0','0','0.96875';'MRR_ObjObstacleProb_22','126','5','BE','unsigned','Standard','0','0.03125','0','0','0.96875';'MRR_ObjRelAccelX_21','72','10','BE','unsigned','Standard','0','0.03125','-16','-16','15.9688';'MRR_ObjRelAccelX_22','176','10','BE','unsigned','Standard','0','0.03125','-16','-16','15.9688';'MRR_ObjRelAccelY_21','94','10','BE','unsigned','Standard','0','0.03125','-16','-16','15.9688';'MRR_ObjRelAccelY_22','198','10','BE','unsigned','Standard','0','0.03125','-16','-16','15.9688';'MRR_ObjRelVelX_21','63','13','BE','unsigned','Standard','0','0.03125','-128','-128','127.9688';'MRR_ObjRelVelX_22','167','13','BE','unsigned','Standard','0','0.03125','-128','-128','127.9688';'MRR_ObjRelVelY_21','66','13','BE','unsigned','Standard','0','0.03125','-128','-128','127.9688';'MRR_ObjRelVelY_22','170','13','BE','unsigned','Standard','0','0.03125','-128','-128','127.9688';'MRR_ObjType_21','90','4','BE','unsigned','Standard','0','1','0','0','15';'MRR_ObjType_22','194','4','BE','unsigned','Standard','0','1','0','0','15';'MRR_ObjUpdFlg_21','100','3','BE','unsigned','Standard','0','1','0','0','7';'MRR_ObjUpdFlg_22','204','3','BE','unsigned','Standard','0','1','0','0','7';'MRR_Obj_21_22_Checksum','248','16','BE','unsigned','Standard','0','1','0','0','65535';'MRR_Obj_21_22_MsgCounter','232','4','BE','unsigned','Standard','0','1','0','0','15'}  IDPort=off  TimestampPort=off  ErrorPort=off  RemotePort=off  LengthPort=off  StatusPort=off  BRSPort=off  ESIPort=off  DLCPort=off  ApplyMinMax=off
      settings: SourceProductBaseCode=ME,XP,VN  DataFormat=CANdb specified signals
  Data Type Conversion{1..6,15..24} (16 alike) : DataTypeConversion  OutDataTypeStr=single  SaturateOnIntegerOverflow=off  RndMeth=Floor
  Data Type Conversion{9..10,13..14,25..28,30} (9 alike) : DataTypeConversion  OutDataTypeStr=int8  SaturateOnIntegerOverflow=off  RndMeth=Floor
  Data Type Conversion{7..8,11..12} (4 alike) : DataTypeConversion  OutDataTypeStr=uint8  SaturateOnIntegerOverflow=off  RndMeth=Floor
  Data Type Conversion29 : DataTypeConversion  OutDataTypeStr=uint16  SaturateOnIntegerOverflow=off  RndMeth=Floor
  VR_ADCU_MRR_Obj_21_22_0x69AFromOutData : Outport  OutDataTypeStr=Bus:VR_ADCU_MRR_Obj_21_22_0x69A
  wires:
  CAN FD Unpack/1 -> Data Type Conversion1/1
  CAN FD Unpack/2 -> Data Type Conversion2/1
  CAN FD Unpack/3 -> Data Type Conversion3/1
  CAN FD Unpack/4 -> Data Type Conversion4/1
  CAN FD Unpack/5 -> Data Type Conversion5/1
  CAN FD Unpack/6 -> Data Type Conversion6/1
  CAN FD Unpack/7 -> Data Type Conversion7/1
  CAN FD Unpack/8 -> Data Type Conversion8/1
  CAN FD Unpack/9 -> Data Type Conversion9/1
  CAN FD Unpack/10 -> Data Type Conversion10/1
  CAN FD Unpack/11 -> Data Type Conversion11/1
  CAN FD Unpack/12 -> Data Type Conversion12/1
  CAN FD Unpack/13 -> Data Type Conversion13/1
  CAN FD Unpack/14 -> Data Type Conversion14/1
  CAN FD Unpack/15 -> Data Type Conversion15/1
  CAN FD Unpack/16 -> Data Type Conversion16/1
  CAN FD Unpack/17 -> Data Type Conversion17/1
  CAN FD Unpack/18 -> Data Type Conversion18/1
  CAN FD Unpack/19 -> Data Type Conversion19/1
  CAN FD Unpack/20 -> Data Type Conversion20/1
  CAN FD Unpack/21 -> Data Type Conversion21/1
  CAN FD Unpack/22 -> Data Type Conversion22/1
  CAN FD Unpack/23 -> Data Type Conversion23/1
  CAN FD Unpack/24 -> Data Type Conversion24/1
  CAN FD Unpack/25 -> Data Type Conversion25/1
  CAN FD Unpack/26 -> Data Type Conversion26/1
  CAN FD Unpack/27 -> Data Type Conversion27/1
  CAN FD Unpack/28 -> Data Type Conversion28/1
  CAN FD Unpack/29 -> Data Type Conversion29/1
  CAN FD Unpack/30 -> Data Type Conversion30/1
  Data Type Conversion1/1 -> Bus Creator/1  "MRR_ObjDistX_21"
  Data Type Conversion2/1 -> Bus Creator/2  "MRR_ObjDistX_22"
  Data Type Conversion3/1 -> Bus Creator/3  "MRR_ObjDistY_21"
  Data Type Conversion4/1 -> Bus Creator/4  "MRR_ObjDistY_22"
  Data Type Conversion5/1 -> Bus Creator/5  "MRR_ObjExistProb_21"
  Data Type Conversion6/1 -> Bus Creator/6  "MRR_ObjExistProb_22"
  Data Type Conversion7/1 -> Bus Creator/7  "MRR_ObjFusionCamID_21"
  Data Type Conversion8/1 -> Bus Creator/8  "MRR_ObjFusionCamID_22"
  Data Type Conversion9/1 -> Bus Creator/9  "MRR_ObjFusionSig_21"
  Data Type Conversion10/1 -> Bus Creator/10  "MRR_ObjFusionSig_22"
  Data Type Conversion11/1 -> Bus Creator/11  "MRR_ObjID_21"
  Data Type Conversion12/1 -> Bus Creator/12  "MRR_ObjID_22"
  Data Type Conversion13/1 -> Bus Creator/13  "MRR_ObjMovingSts_21"
  Data Type Conversion14/1 -> Bus Creator/14  "MRR_ObjMovingSts_22"
  Data Type Conversion15/1 -> Bus Creator/15  "MRR_ObjObstacleProb_21"
  Data Type Conversion16/1 -> Bus Creator/16  "MRR_ObjObstacleProb_22"
  Data Type Conversion17/1 -> Bus Creator/17  "MRR_ObjRelAccelX_21"
  Data Type Conversion18/1 -> Bus Creator/18  "MRR_ObjRelAccelX_22"
  Data Type Conversion19/1 -> Bus Creator/19  "MRR_ObjRelAccelY_21"
  Data Type Conversion20/1 -> Bus Creator/20  "MRR_ObjRelAccelY_22"
  Data Type Conversion21/1 -> Bus Creator/21  "MRR_ObjRelVelX_21"
  Data Type Conversion22/1 -> Bus Creator/22  "MRR_ObjRelVelX_22"
  Data Type Conversion23/1 -> Bus Creator/23  "MRR_ObjRelVelY_21"
  Data Type Conversion24/1 -> Bus Creator/24  "MRR_ObjRelVelY_22"
  Data Type Conversion25/1 -> Bus Creator/25  "MRR_ObjType_21"
  Data Type Conversion26/1 -> Bus Creator/26  "MRR_ObjType_22"
  Data Type Conversion27/1 -> Bus Creator/27  "MRR_ObjUpdFlg_21"
  Data Type Conversion28/1 -> Bus Creator/28  "MRR_ObjUpdFlg_22"
  Data Type Conversion29/1 -> Bus Creator/29  "MRR_Obj_21_22_Checksum"
  Data Type Conversion30/1 -> Bus Creator/30  "MRR_Obj_21_22_MsgCounter"
  Bus Creator/1 -> VR_ADCU_MRR_Obj_21_22_0x69AFromOutData/1  "VR_ADCU_MRR_Obj_21_22_0x69AFromOutData"
  VR_ADCU_MRR_Obj_21_22_0x69AFromInData/1 -> CAN FD Unpack/1  "VR_ADCU_MRR_Obj_21_22_0x69AFromInData"

== system ALL_JP360_DBW_V6_5_1103/MsgFromCAN/VR_ADCU_MsgFromCAN/VR_ADCU_MRR_Obj_23_24_0x69B ==
  VR_ADCU_MRR_Obj_23_24_0x69BFromInData : Inport  OutDataTypeStr=Bus:CAN_FD_MESSAGE_BUS
  Bus Creator : BusCreator  Inputs=30  OutDataTypeStr=Bus:VR_ADCU_MRR_Obj_23_24_0x69B  NonVirtualBus=on
  CAN FD Unpack : canfdmsglib/CAN FD Unpack  CANdbFile=HiFire_T360_P789_1R1V_Pri_Matrix_CAN_V2.3_20220810.dbc  MsgList=(none)  MsgName=MRR_Obj_23_24_0x69B  ProtocolMode=CAN FD  MsgIDType=Standard (11-bit identifier)  MsgIdentifier=1691  MsgLength=32  SignalInfo={'MRR_ObjDistX_23','26','12','BE','unsigned','Standard','0','0.0625','0','0','254.9375';'MRR_ObjDistX_24','130','12','BE','unsigned','Standard','0','0.0625','0','0','254.9375';'MRR_ObjDistY_23','44','14','BE','unsigned','Standard','0','0.0078125','-64','-64','63.9922';'MRR_ObjDistY_24','148','14','BE','unsigned','Standard','0','0.0078125','-64','-64','63.9922';'MRR_ObjExistProb_23','11','5','BE','unsigned','Standard','0','0.03125','0','0','0.96875';'MRR_ObjExistProb_24','115','5','BE','unsigned','Standard','0','0.03125','0','0','0.96875';'MRR_ObjFusionCamID_23','208','8','BE','unsigned','Standard','0','1','0','0','255';'MRR_ObjFusionCamID_24','216','8','BE','unsigned','Standard','0','1','0','0','255';'MRR_ObjFusionSig_23','98','2','BE','unsigned','Standard','0','1','0','0','3';'MRR_ObjFusionSig_24','202','2','BE','unsigned','Standard','0','1','0','0','3';'MRR_ObjID_23','0','8','BE','unsigned','Standard','0','1','0','0','255';'MRR_ObjID_24','104','8','BE','unsigned','Standard','0','1','0','0','255';'MRR_ObjMovingSts_23','103','3','BE','unsigned','Standard','0','1','0','0','7';'MRR_ObjMovingSts_24','207','3','BE','unsigned','Standard','0','1','0','0','7';'MRR_ObjObstacleProb_23','22','5','BE','unsigned','Standard','0','0.03125','0','0','0.96875';'MRR_ObjObstacleProb_24','126','5','BE','unsigned','Standard','0','0.03125','0','0','0.96875';'MRR_ObjRelAccelX_23','72','10','BE','unsigned','Standard','0','0.03125','-16','-16','15.9688';'MRR_ObjRelAccelX_24','176','10','BE','unsigned','Standard','0','0.03125','-16','-16','15.9688';'MRR_ObjRelAccelY_23','94','10','BE','unsigned','Standard','0','0.03125','-16','-16','15.9688';'MRR_ObjRelAccelY_24','198','10','BE','unsigned','Standard','0','0.03125','-16','-16','15.9688';'MRR_ObjRelVelX_23','63','13','BE','unsigned','Standard','0','0.03125','-128','-128','127.9688';'MRR_ObjRelVelX_24','167','13','BE','unsigned','Standard','0','0.03125','-128','-128','127.9688';'MRR_ObjRelVelY_23','66','13','BE','unsigned','Standard','0','0.03125','-128','-128','127.9688';'MRR_ObjRelVelY_24','170','13','BE','unsigned','Standard','0','0.03125','-128','-128','127.9688';'MRR_ObjType_23','90','4','BE','unsigned','Standard','0','1','0','0','15';'MRR_ObjType_24','194','4','BE','unsigned','Standard','0','1','0','0','15';'MRR_ObjUpdFlg_23','100','3','BE','unsigned','Standard','0','1','0','0','7';'MRR_ObjUpdFlg_24','204','3','BE','unsigned','Standard','0','1','0','0','7';'MRR_Obj_23_24_Checksum','248','16','BE','unsigned','Standard','0','1','0','0','65535';'MRR_Obj_23_24_MsgCounter','232','4','BE','unsigned','Standard','0','1','0','0','15'}  IDPort=off  TimestampPort=off  ErrorPort=off  RemotePort=off  LengthPort=off  StatusPort=off  BRSPort=off  ESIPort=off  DLCPort=off  ApplyMinMax=off
      settings: SourceProductBaseCode=ME,XP,VN  DataFormat=CANdb specified signals
  Data Type Conversion{1..6,15..24} (16 alike) : DataTypeConversion  OutDataTypeStr=single  SaturateOnIntegerOverflow=off  RndMeth=Floor
  Data Type Conversion{9..10,13..14,25..28,30} (9 alike) : DataTypeConversion  OutDataTypeStr=int8  SaturateOnIntegerOverflow=off  RndMeth=Floor
  Data Type Conversion{7..8,11..12} (4 alike) : DataTypeConversion  OutDataTypeStr=uint8  SaturateOnIntegerOverflow=off  RndMeth=Floor
  Data Type Conversion29 : DataTypeConversion  OutDataTypeStr=uint16  SaturateOnIntegerOverflow=off  RndMeth=Floor
  VR_ADCU_MRR_Obj_23_24_0x69BFromOutData : Outport  OutDataTypeStr=Bus:VR_ADCU_MRR_Obj_23_24_0x69B
  wires:
  CAN FD Unpack/1 -> Data Type Conversion1/1
  CAN FD Unpack/2 -> Data Type Conversion2/1
  CAN FD Unpack/3 -> Data Type Conversion3/1
  CAN FD Unpack/4 -> Data Type Conversion4/1
  CAN FD Unpack/5 -> Data Type Conversion5/1
  CAN FD Unpack/6 -> Data Type Conversion6/1
  CAN FD Unpack/7 -> Data Type Conversion7/1
  CAN FD Unpack/8 -> Data Type Conversion8/1
  CAN FD Unpack/9 -> Data Type Conversion9/1
  CAN FD Unpack/10 -> Data Type Conversion10/1
  CAN FD Unpack/11 -> Data Type Conversion11/1
  CAN FD Unpack/12 -> Data Type Conversion12/1
  CAN FD Unpack/13 -> Data Type Conversion13/1
  CAN FD Unpack/14 -> Data Type Conversion14/1
  CAN FD Unpack/15 -> Data Type Conversion15/1
  CAN FD Unpack/16 -> Data Type Conversion16/1
  CAN FD Unpack/17 -> Data Type Conversion17/1
  CAN FD Unpack/18 -> Data Type Conversion18/1
  CAN FD Unpack/19 -> Data Type Conversion19/1
  CAN FD Unpack/20 -> Data Type Conversion20/1
  CAN FD Unpack/21 -> Data Type Conversion21/1
  CAN FD Unpack/22 -> Data Type Conversion22/1
  CAN FD Unpack/23 -> Data Type Conversion23/1
  CAN FD Unpack/24 -> Data Type Conversion24/1
  CAN FD Unpack/25 -> Data Type Conversion25/1
  CAN FD Unpack/26 -> Data Type Conversion26/1
  CAN FD Unpack/27 -> Data Type Conversion27/1
  CAN FD Unpack/28 -> Data Type Conversion28/1
  CAN FD Unpack/29 -> Data Type Conversion29/1
  CAN FD Unpack/30 -> Data Type Conversion30/1
  Data Type Conversion1/1 -> Bus Creator/1  "MRR_ObjDistX_23"
  Data Type Conversion2/1 -> Bus Creator/2  "MRR_ObjDistX_24"
  Data Type Conversion3/1 -> Bus Creator/3  "MRR_ObjDistY_23"
  Data Type Conversion4/1 -> Bus Creator/4  "MRR_ObjDistY_24"
  Data Type Conversion5/1 -> Bus Creator/5  "MRR_ObjExistProb_23"
  Data Type Conversion6/1 -> Bus Creator/6  "MRR_ObjExistProb_24"
  Data Type Conversion7/1 -> Bus Creator/7  "MRR_ObjFusionCamID_23"
  Data Type Conversion8/1 -> Bus Creator/8  "MRR_ObjFusionCamID_24"
  Data Type Conversion9/1 -> Bus Creator/9  "MRR_ObjFusionSig_23"
  Data Type Conversion10/1 -> Bus Creator/10  "MRR_ObjFusionSig_24"
  Data Type Conversion11/1 -> Bus Creator/11  "MRR_ObjID_23"
  Data Type Conversion12/1 -> Bus Creator/12  "MRR_ObjID_24"
  Data Type Conversion13/1 -> Bus Creator/13  "MRR_ObjMovingSts_23"
  Data Type Conversion14/1 -> Bus Creator/14  "MRR_ObjMovingSts_24"
  Data Type Conversion15/1 -> Bus Creator/15  "MRR_ObjObstacleProb_23"
  Data Type Conversion16/1 -> Bus Creator/16  "MRR_ObjObstacleProb_24"
  Data Type Conversion17/1 -> Bus Creator/17  "MRR_ObjRelAccelX_23"
  Data Type Conversion18/1 -> Bus Creator/18  "MRR_ObjRelAccelX_24"
  Data Type Conversion19/1 -> Bus Creator/19  "MRR_ObjRelAccelY_23"
  Data Type Conversion20/1 -> Bus Creator/20  "MRR_ObjRelAccelY_24"
  Data Type Conversion21/1 -> Bus Creator/21  "MRR_ObjRelVelX_23"
  Data Type Conversion22/1 -> Bus Creator/22  "MRR_ObjRelVelX_24"
  Data Type Conversion23/1 -> Bus Creator/23  "MRR_ObjRelVelY_23"
  Data Type Conversion24/1 -> Bus Creator/24  "MRR_ObjRelVelY_24"
  Data Type Conversion25/1 -> Bus Creator/25  "MRR_ObjType_23"
  Data Type Conversion26/1 -> Bus Creator/26  "MRR_ObjType_24"
  Data Type Conversion27/1 -> Bus Creator/27  "MRR_ObjUpdFlg_23"
  Data Type Conversion28/1 -> Bus Creator/28  "MRR_ObjUpdFlg_24"
  Data Type Conversion29/1 -> Bus Creator/29  "MRR_Obj_23_24_Checksum"
  Data Type Conversion30/1 -> Bus Creator/30  "MRR_Obj_23_24_MsgCounter"
  Bus Creator/1 -> VR_ADCU_MRR_Obj_23_24_0x69BFromOutData/1  "VR_ADCU_MRR_Obj_23_24_0x69BFromOutData"
  VR_ADCU_MRR_Obj_23_24_0x69BFromInData/1 -> CAN FD Unpack/1  "VR_ADCU_MRR_Obj_23_24_0x69BFromInData"
